simulink model "PNEUMA"  (R2023b)
settings: Solver=ode23tb  StartTime=0  StopTime=3600  FixedStep=0.001  MaxStep=time_step_new  RelTol=0.01  EnableMultiTasking=on
values from neighbouring files (symbols this model uses):
  A = 20.9    [Gas_Exchange_IC.m]    (also in getPneumonia.m = (LF1-LF2)/(1-exp(Rresolve*(t2(end)-t2(1)))))
  a1 = 0.3836    [Dissociation_Spencer_IC.m]    (also in Gas_Exchange_IC.m; Respiratory_IC.m)
  a2 = 1.819    [Dissociation_Spencer_IC.m]    (also in Gas_Exchange_IC.m; Respiratory_IC.m)
  alpha1 = 0.02598    [Dissociation_Spencer_IC.m]    (also in Gas_Exchange_IC.m; Respiratory_IC.m)
  alpha2 = 0.05591    [Dissociation_Spencer_IC.m]    (also in Gas_Exchange_IC.m; Respiratory_IC.m)
  B = 92.8    [Gas_Exchange_IC.m]    (also in getPneumonia.m = LungFunction(end)-A)
  beta1 = 0.012275    [Dissociation_Spencer_IC.m]    (also in Gas_Exchange_IC.m; Respiratory_IC.m)
  beta2 = 0.03255    [Dissociation_Spencer_IC.m]    (also in Gas_Exchange_IC.m; Respiratory_IC.m)
  C = 10570    [Gas_Exchange_IC.m]
  C1 = 9    [Dissociation_Spencer_IC.m]    (also in Gas_Exchange_IC.m; Respiratory_IC.m)
  C2 = 87.00    (= 87)    [Dissociation_Spencer_IC.m]    (also in Gas_Exchange_IC.m; Respiratory_IC.m)
  Circadian_Period = 24    [Respiratory_IC.m]    (also in State_UA_Khoo_IC.m)
  CvCO2IC = 0.5116    [Body_Khoo_IC.m]    (also in Gas_Exchange_IC.m; Respiratory_IC.m = 0.5247)
  CvO2IC = 0.1672    [Body_Khoo_IC.m]    (also in Gas_Exchange_IC.m; Respiratory_IC.m = 0.1639)
  D = -5.251    [Gas_Exchange_IC.m]
  Dead1CO2IC = 0.1020    (= 0.102)    [Dead_Space_Khoo_IC.m]    (also in Gas_Exchange_IC.m; Respiratory_IC.m = 39.5616)
  Dead1O2IC = 149.8824    [Dead_Space_Khoo_IC.m]    (also in Gas_Exchange_IC.m; Respiratory_IC.m = 104.3637)
  Dead2CO2IC = 0.5274    [Dead_Space_Khoo_IC.m]    (also in Gas_Exchange_IC.m; Respiratory_IC.m = 39.6736)
  Dead2O2IC = 149.3923    [Dead_Space_Khoo_IC.m]    (also in Gas_Exchange_IC.m; Respiratory_IC.m = 104.2258)
  Dead3CO2IC = 2.2996    [Dead_Space_Khoo_IC.m]    (also in Gas_Exchange_IC.m; Respiratory_IC.m = 39.8127)
  Dead3O2IC = 147.3503    [Dead_Space_Khoo_IC.m]    (also in Gas_Exchange_IC.m; Respiratory_IC.m = 104.0505)
  Dead4CO2IC = 8.2293    [Dead_Space_Khoo_IC.m]    (also in Gas_Exchange_IC.m; Respiratory_IC.m = 40.0061)
  Dead4O2IC = 140.5179    [Dead_Space_Khoo_IC.m]    (also in Gas_Exchange_IC.m; Respiratory_IC.m = 103.8005)
  Dead5CO2IC = 22.0757    [Dead_Space_Khoo_IC.m]    (also in Gas_Exchange_IC.m; Respiratory_IC.m = 40.3359)
  Dead5O2IC = 124.5641    [Dead_Space_Khoo_IC.m]    (also in Gas_Exchange_IC.m; Respiratory_IC.m = 103.3579)
  DtotalIC = 0.3    [NeuroMuscular_IC.m]    (also in Respiratory_IC.m = 0.32)
  E_CW = 5    [Pleural_Schuessler_IC.m]    (also in Pmus_Flow_Younes_IC.m; Resp_Mech_IC.m; Respiratory_IC.m)
  E_L = 5    [Pleural_Schuessler_IC.m]    (also in Pmus_Flow_Younes_IC.m; Resp_Mech_IC.m; Respiratory_IC.m)
  fc = 0.4/60    (= 0.00666666666667)    [Respiratory_IC.m]    (also in State_UA_Khoo_IC.m)
  fcs_max = 47.78    [Cardiovascular_IC.m]    (also in Reflex_Ursino_IC.m)
  fcs_min = 2.52    [Cardiovascular_IC.m]    (also in Reflex_Ursino_IC.m)
  fcs_zero = 25    [Respiratory_IC.m]
  FlowIC = 0    [Pmus_Flow_Younes_IC.m]    (also in Resp_Mech_IC.m; Respiratory_IC.m)
  fp_inf = 6.3    [Respiratory_IC.m]
  fp_zero = 3.2    [Respiratory_IC.m]
  fs_inf = 2.10    (= 2.1)    [Respiratory_IC.m]
  fs_zero = 16.11    [Respiratory_IC.m]
  ftbs_min = 0.1    [Cardiovascular_IC.m]    (also in SA_Node_Ursino_IC.m)
  gc = 0.008/60    (= 0.000133333333333)    [Respiratory_IC.m]    (also in State_UA_Khoo_IC.m)
  h = 0.0183    [Brain_Khoo_IC.m]    (also in Gas_Exchange_IC.m; Respiratory_IC.m)
  HP_basal = 0.58    [Cardiovascular_IC.m]    (also in SA_Node_Ursino_IC.m)
  Ic = 45    [Gas_Exchange_IC.m]    (also in Respiratory_IC.m; Vent_Drive_Khoo_IC.m)
  IpCO2 = 38    [Gas_Exchange_IC.m]    (also in Respiratory_IC.m; Vent_Drive_Khoo_IC.m)
  IpO2 = 102.4    [Gas_Exchange_IC.m]    (also in Respiratory_IC.m; Vent_Drive_Khoo_IC.m)
  K1 = 13    [Dissociation_Spencer_IC.m]    (also in Gas_Exchange_IC.m; Respiratory_IC.m)
  K2 = 194.4    [Dissociation_Spencer_IC.m]    (also in Gas_Exchange_IC.m; Respiratory_IC.m)
  k_cs = 11.758    [Cardiovascular_IC.m]    (also in Reflex_Ursino_IC.m)
  k_p = 7.06    [Respiratory_IC.m]
  k_s = 0.07    [Respiratory_IC.m]
  lambda = 863    [Gas_Exchange_IC.m]    (also in Lungs_Khoo_IC.m; Respiratory_IC.m)
  Mech_Vent_pressure = 17    [Mech_vent_test.m]
  MRbCO2 = 0.0517    [Brain_Khoo_IC.m]    (also in Gas_Exchange_IC.m; Respiratory_IC.m)
  MRCO2 = 0.0033    [Body_Khoo_IC.m]    (also in Gas_Exchange_IC.m; Respiratory_IC.m)
  MRO2 = 0.0038    [Body_Khoo_IC.m]    (also in Gas_Exchange_IC.m; Respiratory_IC.m)
  NM_block_gain = 1    [Mech_vent_test.m]
  PACO2_delayIC = 39.6041    [Cardio_Mix_Lange_IC.m]    (also in Gas_Exchange_IC.m; Respiratory_IC.m = 40.4448)
  PaCO2firstIC = 0.2150    (= 0.215)    [Cardio_Mix_Lange_IC.m]    (also in Gas_Exchange_IC.m; Respiratory_IC.m = -0.2465)
  PACO2IC = 37.1484    [Gas_Exchange_IC.m]    (also in Lungs_Khoo_IC.m; Respiratory_IC.m = 40.9432)
  PaCO2secondIC = 38.4577    [Cardio_Mix_Lange_IC.m]    (also in Gas_Exchange_IC.m; Respiratory_IC.m = 40.3928)
  PAO2_delayIC = 103.8436    [Cardio_Mix_Lange_IC.m]    (also in Gas_Exchange_IC.m; Respiratory_IC.m = 103.1223)
  PaO2firstIC = -0.2838    [Cardio_Mix_Lange_IC.m]    (also in Gas_Exchange_IC.m; Respiratory_IC.m = 0.3557)
  PAO2IC = 107.1983    [Gas_Exchange_IC.m]    (also in Lungs_Khoo_IC.m; Respiratory_IC.m = 102.5153)
  PaO2secondIC = 105.4828    [Cardio_Mix_Lange_IC.m]    (also in Gas_Exchange_IC.m; Respiratory_IC.m = 103.1435)
  PbCO2IC = 48.2858    [Brain_Khoo_IC.m]    (also in Gas_Exchange_IC.m; Respiratory_IC.m = 48.5383)
  PICO2 = 0    [Dead_Space_Khoo_IC.m]    (also in Gas_Exchange_IC.m; Respiratory_IC.m)
  PIO2 = 150    [Dead_Space_Khoo_IC.m]    (also in Gas_Exchange_IC.m; Respiratory_IC.m)
  PIO2_change = -90    [Mech_vent_test.m]    (also in Respiratory_IC.m = 0)
  Pn = 90    [Cardiovascular_IC.m]    (also in Reflex_Ursino_IC.m)
  Pt_frcIC1 = 0    [Pmus_Flow_Younes_IC.m]    (also in Resp_Mech_IC.m; Respiratory_IC.m)
  Pt_frcIC2 = 0    [Pmus_Flow_Younes_IC.m]    (also in Resp_Mech_IC.m; Respiratory_IC.m)
  QdBo = 0.8333    [Brain_Khoo_IC.m]    (also in Gas_Exchange_IC.m; Respiratory_IC.m)
  R_AW = 1.27    [Pleural_Schuessler_IC.m]    (also in Pmus_Flow_Younes_IC.m; Resp_Mech_IC.m; Respiratory_IC.m)
  R_CW = 1.03    [Pleural_Schuessler_IC.m]    (also in Pmus_Flow_Younes_IC.m; Resp_Mech_IC.m; Respiratory_IC.m)
  R_L = 1.69    [Pleural_Schuessler_IC.m]    (also in Pmus_Flow_Younes_IC.m; Resp_Mech_IC.m; Respiratory_IC.m)
  RC = 0.06    [Pleural_Schuessler_IC.m]    (also in Pmus_Flow_Younes_IC.m; Resp_Mech_IC.m; Respiratory_IC.m)
  rc = 0.2/60    (= 0.00333333333333)    [Respiratory_IC.m]    (also in State_UA_Khoo_IC.m)
  SbCO2 = 0.3600    (= 0.36)    [Brain_Khoo_IC.m]    (also in Gas_Exchange_IC.m; Respiratory_IC.m)
  SCO2 = 0.0043    [Brain_Khoo_IC.m]    (also in Gas_Exchange_IC.m; Respiratory_IC.m)
  SWAo = 0.007    [Respiratory_IC.m]    (also in State_UA_Khoo_IC.m)
  T1 = 1    [Cardio_Mix_Lange_IC.m]    (also in Gas_Exchange_IC.m; Respiratory_IC.m)
  T2 = 2    [Cardio_Mix_Lange_IC.m]    (also in Gas_Exchange_IC.m; Respiratory_IC.m)
  t_end_new = 4*24*60*60    (= 345600)    [Mech_vent_test.m]
  t_end_UA = 0    [Respiratory_IC.m]    (also in State_UA_Khoo_IC.m)
  t_Mech_Vent_duration = 0    [Mech_vent_test.m]
  t_Mech_Vent_start = 0    [Mech_vent_test.m]
  t_Mueller_duration = 0    [NeuroMuscular_IC.m]
  t_Mueller_insp = 0    [NeuroMuscular_IC.m]
  t_Mueller_start = 0    [NeuroMuscular_IC.m]
  t_NM_block_duration = 0    [Mech_vent_test.m]
  t_NM_block_start = 0    [Mech_vent_test.m]
  t_O2_duration = 0    [Mech_vent_test.m]    (also in Respiratory_IC.m)
  t_O2_start = 0    [Mech_vent_test.m]    (also in Respiratory_IC.m)
  t_start_new = 0    [Mech_vent_test.m]
  t_start_UA = 0    [Respiratory_IC.m]    (also in State_UA_Khoo_IC.m)
  t_valsalva_duration = 0    [NeuroMuscular_IC.m]
  t_valsalva_insp = 0    [NeuroMuscular_IC.m]
  t_valsalva_start = 0    [NeuroMuscular_IC.m]
  time_step = time_step    [acquire_data.m]    (also in acquire_data_save.m)
  VC = 5    [Pmus_Flow_Younes_IC.m]    (also in Resp_Mech_IC.m; Respiratory_IC.m)
  Vdead1 = 0.03    [Dead_Space_Khoo_IC.m]    (also in Gas_Exchange_IC.m; Respiratory_IC.m)
  Vdead2 = 0.03    [Dead_Space_Khoo_IC.m]    (also in Gas_Exchange_IC.m; Respiratory_IC.m)
  Vdead3 = 0.03    [Dead_Space_Khoo_IC.m]    (also in Gas_Exchange_IC.m; Respiratory_IC.m)
  Vdead4 = 0.03    [Dead_Space_Khoo_IC.m]    (also in Gas_Exchange_IC.m; Respiratory_IC.m)
  Vdead5 = 0.03    [Dead_Space_Khoo_IC.m]    (also in Gas_Exchange_IC.m; Respiratory_IC.m)
  Ventilator_rate = 12    [Mech_vent_test.m]
  VTCO2 = 15    [Body_Khoo_IC.m]    (also in Gas_Exchange_IC.m; Respiratory_IC.m)
  VtIC = 0    [Pmus_Flow_Younes_IC.m]    (also in Resp_Mech_IC.m; Respiratory_IC.m)
  VTO2 = 6    [Body_Khoo_IC.m]    (also in Gas_Exchange_IC.m; Respiratory_IC.m)
  Z = 0.0227    [Dissociation_Spencer_IC.m]    (also in Gas_Exchange_IC.m; Respiratory_IC.m)
undefined symbols (not defined in the file or in its folder): A_0_ua, alpha_E_FFA_Heart, alpha_E_FFA_muscle, alpha_E_GLC_Heart, alpha_E_GLC_muscle, alpha_E_GLY_muscle, alpha_E_PYR_muscle, alpha_E_TGL_adipose, alpha_E_TGL_GI, alpha_E_TGL_Heart, alpha_E_TGL_muscle, Arousal_UAIC, C_ua_awake, Cbp, Cbv, Ce_0, Cep, Cev, Chp, Chv, Cla, Clamp_class, Cmp, Cmv, Cpa, CPAP_pressure, Cpp, Cpv, Cra, Csa, Csp, Csv, CvbO2_n, CvhO2_n, CvmO2_n, DAY, delay, DietBlock, Dx, Fb, fchemo_max, fchemo_min, fchemoIC, flsIC, Ftas_I0, ftas_min, ftas_r0, FVC_activation, gain_E, Gamma, Gas_sleep, Gas_sleepM, Gb, Gblock, GbO2, Gbs_sleep, gcc_sa, gcc_sb, gcc_sp, Gclamp ... (+144)
libraries: simulink x4, dspstat3 x4, simulink_extras x2
(part 3 of 8)

== system PNEUMA/FVC + Valsalva + Mueller maneuvers/MEFV Operation ==
  Fcn1 : Fcn  Expr=1-u
  Mux2 : Mux  Inputs=3
  Step : Step  Time=begin_time  SampleTime=0
  Step1 : Step  Time=begin_time+duration_time  After=-1  SampleTime=0
  Step3 : Step  Time=begin_time+insp_period  After=-1  SampleTime=0
  Step5 : Step  Time=begin_time+insp_period  After=-1  SampleTime=0
  Step7 : Step  Time=begin_time+0.01  After=-1  SampleTime=0
  Step8 : Step  Time=begin_time+insp_period  SampleTime=0
  Step9 : Step  Time=begin_time+duration_time  After=-1  SampleTime=0
  Sum{,1..4} (5 alike) : Sum  Inputs=|++  InputSameDT=on  SaturateOnIntegerOverflow=on  OutDataTypeStr=Inherit: Same as first input
  duration : Outport
  FVC_rhythm : Outport  Port=2
  FVC_resp_mech : Outport  Port=3
  wires:
  Fcn1/1 -> duration/1
  Sum4/1 -> FVC_resp_mech/1
  Step8/1 -> Sum4/1
  Mux2/1 -> FVC_rhythm/1
  Sum3/1 -> Mux2/3
  Step7/1 -> Sum3/2
  Sum2/1 -> Mux2/2
  Step5/1 -> Sum2/2
  Sum1/1 -> Mux2/1
  Step3/1 -> Sum1/2
  Sum/1 -> Fcn1/1
  Step1/1 -> Sum/2
  Step/1 -> Sum/1, Sum1/1, Sum2/1, Sum3/1
  Step9/1 -> Sum4/2

== system PNEUMA/FVC + Valsalva + Mueller maneuvers/Mueller Operation ==
  Fcn1 : Fcn  Expr=1-u
  Fcn2 : Fcn  Expr=1-u
  Mux2 : Mux  Inputs=3
  Step : Step  Time=begin_time  SampleTime=0
  Step1 : Step  Time=begin_time+duration_time  After=-1  SampleTime=0
  Step3 : Step  Time=begin_time+insp_period  After=-1  SampleTime=0
  Step5 : Step  Time=begin_time+insp_period  After=-1  SampleTime=0
  Step7 : Step  Time=begin_time+0.01  After=-1  SampleTime=0
  Step9 : Step  Time=begin_time+insp_period+0.5  After=-1  SampleTime=0
  Sum{,1..4} (5 alike) : Sum  Inputs=|++  InputSameDT=on  SaturateOnIntegerOverflow=on  OutDataTypeStr=Inherit: Same as first input
  duration : Outport
  mueller_rhythm : Outport  Port=2
  muller_resp_mech : Outport  Port=3
  wires:
  Fcn2/1 -> muller_resp_mech/1
  Fcn1/1 -> duration/1
  Step/1 -> Sum/1, Sum1/1, Sum2/1, Sum3/1, Sum4/1
  Step1/1 -> Sum/2
  Sum/1 -> Fcn1/1
  Step3/1 -> Sum1/2
  Sum1/1 -> Mux2/1
  Step5/1 -> Sum2/2
  Sum2/1 -> Mux2/2
  Step7/1 -> Sum3/2
  Sum3/1 -> Mux2/3
  Mux2/1 -> mueller_rhythm/1
  Step9/1 -> Sum4/2
  Sum4/1 -> Fcn2/1

== system PNEUMA/FVC + Valsalva + Mueller maneuvers/Valsalva Operation ==
  Fcn1 : Fcn  Expr=1-u
  Mux2 : Mux  Inputs=3
  Step : Step  Time=begin_time  SampleTime=0
  Step1 -(TTmean-TImean) : Step  Time=begin_time+duration_time  After=-1  SampleTime=0
  Step3 : Step  Time=begin_time+insp_period  After=-1  SampleTime=0
  Step5 : Step  Time=begin_time+insp_period  After=-1  SampleTime=0
  Step7 : Step  Time=begin_time+0.01  After=-1  SampleTime=0
  Step8 : Step  Time=begin_time+insp_period  SampleTime=0
  Step9 : Step  Time=begin_time+duration_time  After=-1  SampleTime=0
  Sum{,1..4} (5 alike) : Sum  Inputs=|++  InputSameDT=on  SaturateOnIntegerOverflow=on  OutDataTypeStr=Inherit: Same as first input
  duration : Outport
  valsalva_rhythm : Outport  Port=2
  valsalva_resp_mech : Outport  Port=3
  wires:
  Fcn1/1 -> duration/1
  Sum4/1 -> valsalva_resp_mech/1
  Step8/1 -> Sum4/1
  Mux2/1 -> valsalva_rhythm/1
  Sum3/1 -> Mux2/3
  Step7/1 -> Sum3/2
  Sum2/1 -> Mux2/2
  Step5/1 -> Sum2/2
  Sum1/1 -> Mux2/1
  Step3/1 -> Sum1/2
  Sum/1 -> Fcn1/1
  Step1 -(TTmean-TImean)/1 -> Sum/2
  Step/1 -> Sum/1, Sum1/1, Sum2/1, Sum3/1
  Step9/1 -> Sum4/2

== system PNEUMA/Metabolic Control/Display & Storage ==
  note: Sample Rate: Default
  I(t)_in : Inport
  G(t) : Inport  Port=2
  I(t) : Inport  Port=3
  F(t) : Inport  Port=4
  E(t) : Inport  Port=5
  Gin : Inport  Port=6
  Gclamp_in : Inport  Port=7
  Main Display : Scope  NumInputPorts=6
  Mux : Mux  Inputs=7
  Saving G_I_FFA : Subsystem
  tag scope: Epinephrine=global, FFA=global, Glucose=global, GlucoseInput=global, Insulin=global
  wires:
  G(t)/1 -> Main Display/1, Mux/1, [Glucose]
  I(t)/1 -> Main Display/2, Mux/2, [Insulin]
  F(t)/1 -> Mux/3, Main Display/3, [FFA]
  E(t)/1 -> Mux/4, Main Display/4, [Epinephrine]
  Gin/1 -> Mux/5, [GlucoseInput], Main Display/5
  I(t)_in/1 -> Mux/6
  Mux/1 -> Saving G_I_FFA/1(In1)
  Gclamp_in/1 -> Main Display/6, Mux/7

== system PNEUMA/Metabolic Control/Epinephrine Regulation on Heart and Muscle ==
  note: (micronmol/min)
  note: (micronmol/min)
  note: (micronmol/min)
  Ftas_r : Inport
  SI : Inport  Port=2
  REM : Inport  Port=3
  1microMol = 1e6 pMol : Gain  Gain=1e6  SaturateOnIntegerOverflow=on  OutDataTypeStr=Inherit: Same as input  ParamDataTypeStr=Inherit: Same as input
  Demux : Demux
  Demux1 : Demux  Outputs=5
  EPI Modulation : Scope  NumInputPorts=10
  Epi Dynamics : Subsystem
  Epi Modulation : Subsystem
  FLux Scope : Scope  NumInputPorts=4
  Subtract : Sum  Inputs=-+
  Subtract1 : Sum  Inputs=-+
  "Epi_Heart Glucose " : Outport
  Epi_Muscle Glucose : Outport  Port=2
  "Epi_Heart FFA " : Outport  Port=3
  Epi_Muscle FFA : Outport  Port=4
  Epi_GI FFA : Outport  Port=5
  Epinephrine Amount Ce(t) : Outport  Port=6
  W_alphaSYMP : Outport  Port=7
  wires:
  Epi Dynamics/1(Ce(t)) -> 1microMol = 1e6 pMol/1
  Epi Modulation/1(Epi on Heart) -> FLux Scope/1
  Epi Modulation/2(Epi on Muscle) -> FLux Scope/2
  Epi Modulation/3(Epi on GI) -> FLux Scope/3, EPI Modulation/10, Epi_GI FFA/1
  Epi Modulation/4(Epi on adipose) -> FLux Scope/4
  1microMol = 1e6 pMol/1 -> Epi Modulation/1(Ce(t)), Epinephrine Amount Ce(t)/1
  Epi Modulation/5(4Fluxes of Epi in Heart) -> Demux/1
  Epi Modulation/6(5Fluxes of Epi in Muscle) -> Demux1/1
  Demux/1 -> EPI Modulation/1, "Epi_Heart Glucose "/1
  Demux/2 -> EPI Modulation/2
  Demux/3 -> EPI Modulation/3, Subtract/1
  Demux/4 -> EPI Modulation/4, Subtract/2
  Demux1/1 -> EPI Modulation/5, Epi_Muscle Glucose/1
  Demux1/2 -> EPI Modulation/6
  Demux1/3 -> EPI Modulation/7
  Demux1/4 -> EPI Modulation/8, Subtract1/1
  Demux1/5 -> EPI Modulation/9, Subtract1/2
  Subtract/1 -> "Epi_Heart FFA "/1
  Subtract1/1 -> Epi_Muscle FFA/1
  Ftas_r/1 -> Epi Dynamics/1(Ftas_r)
  SI/1 -> Epi Dynamics/2(SI)
  REM/1 -> Epi Dynamics/3(REM)
  Epi Dynamics/2(W_alphaSYMP) -> W_alphaSYMP/1

== system PNEUMA/Metabolic Control/Gain ==
  In1 : Inport
  In2 : Inport  Port=2
  In3 : Inport  Port=3
  In4 : Inport  Port=4
  In5 : Inport  Port=5
  Subtract1 : Sum
  Subtract2 : Sum  Inputs=+++
  micromol to mg : Gain  Gain=0.0018*gain_E
  micromol to mg1 : Gain  Gain=0.01*gain_E
  G_E : Outport
  F_E : Outport  Port=2
  wires:
  Subtract1/1 -> micromol to mg/1  "Glucose Input"
  Subtract2/1 -> micromol to mg1/1  "FFA Input"
  In1/1 -> Subtract1/1
  micromol to mg/1 -> G_E/1  "Glucose Input"
  In2/1 -> Subtract1/2
  In3/1 -> Subtract2/1
  In4/1 -> Subtract2/2
  micromol to mg1/1 -> F_E/1
  In5/1 -> Subtract2/3

== system PNEUMA/Metabolic Control/Glucose Insulin Interventions ==
  note: 1-IVGTT (1hr only)
      | 2-Glucose Clamps
  G(t) : Inport
  1-Hyper&2-Norm_Hypo : Constant  Value=Clamp_class
  GI_CTRL : Constant  Value=GI_CTRL
  Gblock : Gain  Gain=0
  Hyper/Eu/Hypo glycemic Clamp (step by step) : Subsystem
  IVGTT : Subsystem  mask{begin_time=0, end_time=1*60, init_value=330*70/70, end_value=0}
      mask prompts: begin_time "begin time"; end_time "end time"; init_value "initial value"; end_value "end value"
      mask Display: disp('IVGTT')
  Iblock : Gain  Gain=0
  Insulin Pump Euglycemic Clamp : Subsystem
  Multiport Switch : MultiPortSwitch  Inputs=2  SaturateOnIntegerOverflow=off  InputSameDT=off
  Glu_in(t) : Outport
  Gclamp_in(t) : Outport  Port=2
  InsPump_in(t) : Outport  Port=3
  wires:
  IVGTT/1(Out1) -> Multiport Switch/2
  Multiport Switch/1 -> Gblock/1
  GI_CTRL/1 -> Multiport Switch/1
  Insulin Pump Euglycemic Clamp/1(Out1) -> Iblock/1
  Hyper/Eu/Hypo glycemic Clamp (step by step)/1(u(t)) -> Multiport Switch/3
  1-Hyper&2-Norm_Hypo/1 -> Hyper/Eu/Hypo glycemic Clamp (step by step)/2(Clamp Classifier)
  G(t)/1 -> Hyper/Eu/Hypo glycemic Clamp (step by step)/1(G(t))
  Gblock/1 -> Glu_in(t)/1
  Hyper/Eu/Hypo glycemic Clamp (step by step)/2(Glu_In Rate) -> Gclamp_in(t)/1
  Iblock/1 -> InsPump_in(t)/1

== system PNEUMA/Metabolic Control/Glucose-Insulin-FFA Minimal Model ==
  note: Remote
      | Insulin
      | X(t)
  u1(t) : Inport
  u2(t) : Inport  Port=2
  u3(t) : Inport  Port=3
  W_alphaSYMP : Inport  Port=4
  2*Fcn+2 : Fcn  Expr=2*Ftas_I0* ( exp((u-Ib)/k_isc_I) -1) / (1+ exp((u-Ib)/k_isc_I) )+2
  FFA Dynamics_LC : Subsystem
  Gain1 : Gain  Gain=1/tao_I
  Glucose Dynamics_LC : Subsystem
  Insulin Dynamics _ B&P : Subsystem
  Integrator1 : Integrator
  Mux : Mux  Inputs=2
  Remote Compartment p3 / (s + p2)1 : Subsystem
  Remote Ins_FFA pF3 / (s + pF2) : Subsystem
  Saving deltaFtas_WalphaSYMP : Subsystem
  Subsystem : Subsystem
  Sum2 : Sum  Inputs=-+  InputSameDT=on  SaturateOnIntegerOverflow=on  OutDataTypeStr=Inherit: Same as first input
  "Plasma Glucose Concn, G(t)" : Outport
  "Plasma Insulin Concn, I(t)" : Outport  Port=2
  "Plasma FFA Concn, F(t)" : Outport  Port=3
  DeltaFtas : Outport  Port=4
  wires:
  Remote Compartment p3 / (s + p2)1/1(X(t)) -> Glucose Dynamics_LC/3(X(t))
  u3(t)/1 -> FFA Dynamics_LC/3(u3(t))
  u2(t)/1 -> Glucose Dynamics_LC/1(u2(t))
  u1(t)/1 -> Insulin Dynamics _ B&P/2(u1(t))
  FFA Dynamics_LC/1(F(t)) -> "Plasma FFA Concn, F(t)"/1, Subsystem/1(F(t))
  Subsystem/1(Z(t)) -> Glucose Dynamics_LC/2(Z(t))  "Remote FFA  Z(t)"
  Insulin Dynamics _ B&P/1(I(t)) -> "Plasma Insulin Concn, I(t)"/1, 2*Fcn+2/1, Remote Compartment p3 / (s + p2)1/1(I(t)), Remote Ins_FFA pF3 / (s + pF2)/1(I(t))
  Remote Ins_FFA pF3 / (s + pF2)/1(Y(t)) -> FFA Dynamics_LC/2(Y(t))
  Sum2/1 -> Gain1/1
  Integrator1/1 -> Sum2/1, Mux/1, DeltaFtas/1
  Gain1/1 -> Integrator1/1
  2*Fcn+2/1 -> Sum2/2
  Glucose Dynamics_LC/1(G(t)) -> "Plasma Glucose Concn, G(t)"/1, Insulin Dynamics _ B&P/1(G(t)), FFA Dynamics_LC/1(G(t))
  W_alphaSYMP/1 -> Mux/2
  Mux/1 -> Saving deltaFtas_WalphaSYMP/1(In1)

== system PNEUMA/Metabolic Control/Insulin Clamp ==
  note: 90-minute Insulin Pump (through 4 steps injections)
  Add : Sum  Inputs=+++++
  Step : Step  Time=2*60+delay+60*2*60  After=step_u1  SampleTime=0
  Step1 : Step  Time=4*60+delay+60*2*60  After=step_u1  SampleTime=0
  Step2 : Step  Time=6*60+delay+60*2*60  After=step_u1  SampleTime=0
  Step3 : Step  Time=8*60+delay+60*2*60  After=step_u1  SampleTime=0
  Step4 : Step  Time=90*60+delay+60*2*60  After=-4*step_u1*Ins_shutdown  SampleTime=0
  Insulin Input : Outport
  wires:
  Step/1 -> Add/1
  Step1/1 -> Add/2
  Step3/1 -> Add/4
  Step2/1 -> Add/3
  Add/1 -> Insulin Input/1
  Step4/1 -> Add/5

== system PNEUMA/Respiratory System/Gas Exchange ==
  Vt - Tidal Volume : Inport
  SI Sleep Wake State Index : Inport  Port=2
  Air Flow : Inport  Port=3
  Blood Flow : Inport  Port=4
  BODY TISSUES COMPARTMENT : Subsystem
  BRAIN COMPARTMENT : Subsystem
  Blood Flow to Tissues : Gain  Gain=0.85  SaturateOnIntegerOverflow=on  OutDataTypeStr=Inherit: Same as input  ParamDataTypeStr=Inherit: Same as input
  Cardiovascular Mixing and Convection : Subsystem
  DEAD SPACE : Subsystem
  Dissociation : Subsystem
  GAS EXCHANGE IN THE LUNGS : Subsystem
  Lung-Chemo Volume : Constant  Value=0.588
  VARIATION OF CEREBRAL BLOOD FLOW W/ PaCO2 Fcn : Fcn  Expr=(sqrt(abs( ((1+(u - 40) * .03 ) * (-QdBo))^2 - ( MRbCO2-h) * 4*0.03*QdBo/SCO2 ) )- (1+(u - 40) * .03 ) * (-QdBo)) *0.5
  PaCO2 : Outport
  PaO2 : Outport  Port=2
  SAO2 : Outport  Port=3
  PbCO2 : Outport  Port=4
  CaO2 : Outport  Port=5
  tag scope: PaCO2=global, PaO2=global, SAO2=global
  wires:
  SI Sleep Wake State Index/1 -> BODY TISSUES COMPARTMENT/1(SI Sleep Wake State Index), BRAIN COMPARTMENT/3(SI Sleep Wake State Index)
  Cardiovascular Mixing and Convection/1(PaCO2) -> BRAIN COMPARTMENT/2(PaCO2), [PaCO2], PaCO2/1  "PaCO2"
  BRAIN COMPARTMENT/1(PbCO2) -> PbCO2/1, VARIATION OF CEREBRAL BLOOD FLOW W/ PaCO2 Fcn/1  "PbCO2"
  DEAD SPACE/1(Pd5CO2) -> GAS EXCHANGE IN THE LUNGS/3(Pd5CO2)
  DEAD SPACE/2(Pd5O2) -> GAS EXCHANGE IN THE LUNGS/4(Pd5O2)
  GAS EXCHANGE IN THE LUNGS/2(PAO2) -> DEAD SPACE/2(PAO2), Cardiovascular Mixing and Convection/3(PAO2), Dissociation/2(PAO2)  "PAO2"
  Vt - Tidal Volume/1 -> GAS EXCHANGE IN THE LUNGS/6(Vt - Tidal Volume)
  Air Flow/1 -> DEAD SPACE/3(Flow), GAS EXCHANGE IN THE LUNGS/5(Flow)
  VARIATION OF CEREBRAL BLOOD FLOW W/ PaCO2 Fcn/1 -> BRAIN COMPARTMENT/1(Qb)  "Qb"
  GAS EXCHANGE IN THE LUNGS/1(PACO2) -> DEAD SPACE/1(PACO2), Cardiovascular Mixing and Convection/2(PACO2), Dissociation/1(PACO2)  "PACO2"
  Lung-Chemo Volume/1 -> Cardiovascular Mixing and Convection/1(Lung-Chemoreceptor Delay Volume)
  Blood Flow/1 -> Blood Flow to Tissues/1, GAS EXCHANGE IN THE LUNGS/7("Q "), Cardiovascular Mixing and Convection/4(Q)
  Cardiovascular Mixing and Convection/2(PaO2) -> [PaO2], PaO2/1  "PaO2"
  Blood Flow to Tissues/1 -> BODY TISSUES COMPARTMENT/4("Qt ")
  Dissociation/1(CaCO2) -> GAS EXCHANGE IN THE LUNGS/1(CaCO2), BODY TISSUES COMPARTMENT/2(CaCO2)
  Dissociation/3(CaO2) -> GAS EXCHANGE IN THE LUNGS/9(CaO2), CaO2/1, BODY TISSUES COMPARTMENT/3(CaO2)
  Dissociation/2(SAO2) -> [SAO2], SAO2/1
  BODY TISSUES COMPARTMENT/1(CvCO2) -> GAS EXCHANGE IN THE LUNGS/2(CVCO2)
  BODY TISSUES COMPARTMENT/2(CvO2) -> GAS EXCHANGE IN THE LUNGS/8(CVO2)

== system PNEUMA/Respiratory System/Modified Upper Airway Conductance ==
  Fcn1 : Fcn  Expr=1-u
  Fcn2 : Fcn  Expr=(u(1)==0)*1+(u(1)==1)*u(2)
  Fcn3 : Fcn  Expr=(u(1)==0)*1+(u(1)==1)*u(2)
  Memory : Memory
  Mux1 : Mux  Inputs=2
  Mux3 : Mux  Inputs=2
  Product2 : Product  Inputs=***  InputSameDT=on  SaturateOnIntegerOverflow=on  OutDataTypeStr=Inherit: Same as first input
  Sum : Sum
  Terminator : Terminator
  UA_blocker : Gain  Gain=0  SaturateOnIntegerOverflow=on  OutDataTypeStr=Inherit: Same as input  ParamDataTypeStr=Inherit: Same as input
  UPC Scope : Scope  NumInputPorts=4
  Upper Airway Blockage : Subsystem  mask{begin_time=t_start_UA, end_time=t_end_UA}
      mask prompts: begin_time "pulse begin"; end_time "pulse end"
      mask Display: disp('pulse')
  func : Fcn  Expr=1-u
  modified upper airway : Outport
  tag scope: upper_airway_blockage_duration=global
  wires:
  Upper Airway Blockage/1(Out1) -> func/1
  [Valsalva_resp_mech] -> Fcn1/1
  UA_blocker/1 -> [upper_airway_blockage_duration], Sum/1
  [CONDua] -> Product2/1, UPC Scope/3
  Product2/1 -> UPC Scope/2, Sum/2
  func/1 -> UA_blocker/1
  [Mueller_activation] -> Mux3/1
  [Mueller_resp_mech] -> Mux3/2
  Mux3/1 -> Fcn2/1
  Fcn2/1 -> Product2/2
  [Valsalva_activation] -> Mux1/1
  Mux1/1 -> Fcn3/1
  Fcn1/1 -> Mux1/2
  Fcn3/1 -> UPC Scope/4, Terminator/1, Product2/3
  Memory/1 -> modified upper airway/1, UPC Scope/1
  Sum/1 -> Memory/1

== system PNEUMA/Respiratory System/Respiratory_Mechanics ==
  "RespMus Drive " : Inport
  Respiratory Conductance : Inport  Port=2
  "PE " : Inport  Port=3
  "Pao " : Inport  Port=4
  Step Size : Inport  Port=5
  Enable : EnablePort  StatesWhenEnabling=reset  ZeroCross=off
  External Pressure Gain : Gain  Gain=0.1  SaturateOnIntegerOverflow=on  OutDataTypeStr=Inherit: Same as input  ParamDataTypeStr=Inherit: Same as input
  Pleural Pressure Saturation : Saturate  UpperLimit=160  LowerLimit=-40  LinearizeAsGain=off  ZeroCross=off
  Pleural_Pressure1 : Subsystem
  Respiratory Muscles Activity1 : Subsystem
  Vt - Tidal Volume : Outport  InitialOutput=[0]
  Respiratory Flow : Outport  Port=2  InitialOutput=[0]
  "Ppl " : Outport  Port=3  InitialOutput=[0]
  wires:
  "PE "/1 -> Respiratory Muscles Activity1/2(PE)
  "RespMus Drive "/1 -> Respiratory Muscles Activity1/1(RespMus Drive)
  Respiratory Conductance/1 -> Respiratory Muscles Activity1/3("cond ")
  Respiratory Muscles Activity1/3(Pmus) -> Pleural_Pressure1/3(Pmus)
  "Pao "/1 -> External Pressure Gain/1
  External Pressure Gain/1 -> Pleural_Pressure1/4("Pao "), Respiratory Muscles Activity1/5(Pao)
  Respiratory Muscles Activity1/2(Vt) -> Pleural_Pressure1/2(Vt), Vt - Tidal Volume/1  "Vt Tidal Volume"
  Respiratory Muscles Activity1/1(Respiratory Flow) -> Pleural_Pressure1/1(Respiratory Flow), Respiratory Flow/1  "Flow"
  Step Size/1 -> Respiratory Muscles Activity1/4(Step Size)
  Pleural_Pressure1/1("Pleural Pressure (Ppl) ") -> Pleural Pressure Saturation/1
  Pleural Pressure Saturation/1 -> "Ppl "/1

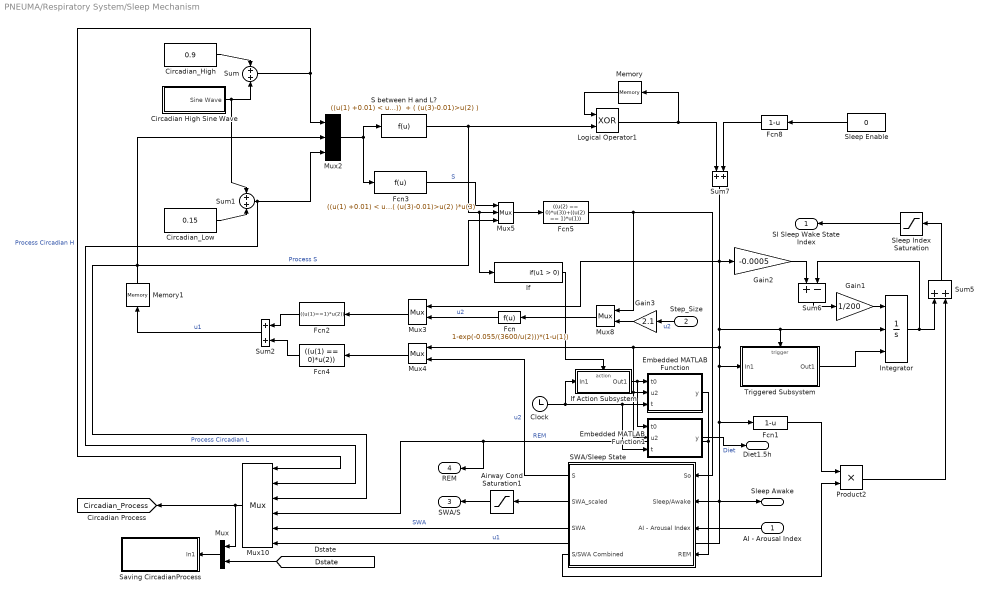
== system PNEUMA/Respiratory System/Sleep Mechanism ==
  AI - Arousal Index : Inport
  Step_Size : Inport  Port=2
  Airway Cond Saturation1 : Saturate  UpperLimit=1  LowerLimit=0
  Circadian High Sine Wave : Subsystem
  Circadian_High : Constant  Value=0.9
  Circadian_Low : Constant  Value=0.15
  Clock : Clock
  Embedded MATLAB Function : MATLAB Function  TreatAsAtomicUnit=on
  Embedded MATLAB Function1 : MATLAB Function  TreatAsAtomicUnit=on
  Fcn : Fcn  Expr=1-exp(-0.055/(3600/u(2)))*(1-u(1))
  Fcn1 : Fcn  Expr=1-u
  Fcn2 : Fcn  Expr=((u(1)==1)*u(2))
  Fcn3 : Fcn  Expr=((u(1) +0.01) < u(2)) * u(1) + ( (u(3)-0.01)>u(2) )*u(3)
  Fcn4 : Fcn  Expr=((u(1) == 0)*u(2))
  Fcn5 : Fcn  Expr=((u(2) == 0)*u(3))+((u(2) == 1)*u(1))
  Fcn8 : Fcn  Expr=1-u
  Gain1 : Gain  Gain=1/200  SaturateOnIntegerOverflow=on  OutDataTypeStr=Inherit: Same as input  ParamDataTypeStr=Inherit: Same as input
  Gain2 : Gain  Gain=-0.0005  SaturateOnIntegerOverflow=on  OutDataTypeStr=Inherit: Same as input  ParamDataTypeStr=Inherit: Same as input
  Gain3 : Gain  Gain=2.1  SaturateOnIntegerOverflow=on  OutDataTypeStr=Inherit: Same as input  ParamDataTypeStr=Inherit: Same as input
  If : If  ShowElse=off
  If Action Subsystem : Subsystem  TreatAsAtomicUnit=on
  Integrator : Integrator  ExternalReset=rising  InitialConditionSource=external  InitialCondition=1
  Logical Operator1 : Logic  Operator=XOR
  Memory : Memory  InitialCondition=1  InheritSampleTime=on
  Memory1 : Memory  InitialCondition=1  InheritSampleTime=on
  Mux{,3..4,8} (4 alike) : Mux  Inputs=2
  Mux10 : Mux  Inputs=6
  Mux2 : Mux  Inputs=3
  Mux5 : Mux  Inputs=3
  Product2 : Product  InputSameDT=on  SaturateOnIntegerOverflow=on  OutDataTypeStr=Inherit: Same as first input
  S between H and L? : Fcn  Expr="((u(1) +0.01) < u(2))  + ( (u(3)-0.01)>u(2) )"
  SWA/Sleep State : Subsystem
  Saving CircadianProcess : Subsystem
  Sleep Enable : Constant  Value=0
  Sleep Index Saturation : Saturate  UpperLimit=1  LowerLimit=0
  Sum{,1..2,5,7} (5 alike) : Sum  InputSameDT=on  SaturateOnIntegerOverflow=on  OutDataTypeStr=Inherit: Same as first input
  Sum6 : Sum  Inputs=+-  InputSameDT=on  SaturateOnIntegerOverflow=on  OutDataTypeStr=Inherit: Same as first input
  Triggered Subsystem : Subsystem  TreatAsAtomicUnit=on
  SI Sleep Wake State Index : Outport
  Sleep Awake : Outport  Port=2
  SWA/S : Outport  Port=3
  REM : Outport  Port=4
  Diet1.5h : Outport  Port=5
  tag scope: Circadian_Process=global
  wires:
  AI - Arousal Index/1 -> SWA/Sleep State/3(AI - Arousal Index)
  Circadian_High/1 -> Sum/1
  Circadian High Sine Wave/1(Sine Wave) -> Sum/2, Sum1/1
  Circadian_Low/1 -> Sum1/2
  Sum/1 -> Mux2/1, Mux10/1  "Process Circadian H"
  Sum1/1 -> Mux2/3, Mux10/2  "Process Circadian L"
  Memory/1 -> Logical Operator1/1
  Logical Operator1/1 -> Memory/1, Sum7/1
  Fcn3/1 -> Mux5/1  "S"
  Fcn2/1 -> Sum2/1
  Sum2/1 -> Memory1/1  "u1"
  Fcn/1 -> Mux3/2  "u2"
  SWA/Sleep State/1(S) -> Mux4/2  "u2"
  Mux5/1 -> Fcn5/1
  Mux3/1 -> Fcn2/1
  Mux4/1 -> Fcn4/1
  Fcn5/1 -> SWA/Sleep State/1(So), Mux8/1
  Mux8/1 -> Fcn/1
  Step_Size/1 -> Gain3/1  "u2"
  SWA/Sleep State/2(SWA_scaled) -> Airway Cond Saturation1/1
  Airway Cond Saturation1/1 -> SWA/S/1
  Mux10/1 -> [Circadian_Process], Mux/1
  SWA/Sleep State/3(SWA) -> Mux10/5  "SWA"
  SWA/Sleep State/4(S/SWA Combined) -> Product2/2
  Fcn1/1 -> Product2/1
  Sum5/1 -> Sleep Index Saturation/1
  Product2/1 -> Sum5/2
  Sleep Index Saturation/1 -> SI Sleep Wake State Index/1
  Sum7/1 -> Mux3/1, Triggered Subsystem/Trigger, Integrator/2, Fcn1/1, Sleep Awake/1, SWA/Sleep State/2(Sleep/Awake), Mux10/6, Triggered Subsystem/1(In1), Mux4/1, Embedded MATLAB Function/2(u2), Embedded MATLAB Function1/2(u2), Gain2/1  "u1"
  Integrator/1 -> Sum5/1, Sum6/2
  Triggered Subsystem/1(Out1) -> Integrator/3
  Gain2/1 -> Sum6/1
  Sum6/1 -> Gain1/1
  Gain1/1 -> Integrator/1
  Fcn8/1 -> Sum7/2
  Memory1/1 -> Mux5/3, Mux10/3, Mux2/2  "Process S"
  Mux2/1 -> Fcn3/1, S between H and L?/1
  S between H and L?/1 -> Logical Operator1/2, Mux5/2, If/1
  Gain3/1 -> Mux8/2
  If Action Subsystem/1(Out1) -> Embedded MATLAB Function/1(t0), Embedded MATLAB Function1/1(t0)
  If/1 -> If Action Subsystem/Action
  Fcn4/1 -> Sum2/2
  Clock/1 -> If Action Subsystem/1(In1), Embedded MATLAB Function/3(t), Embedded MATLAB Function1/3(t)
  Embedded MATLAB Function/1(y) -> SWA/Sleep State/4(REM), Mux10/4, REM/1  "REM"
  Sleep Enable/1 -> Fcn8/1
  [Dstate] -> Mux/2
  Mux/1 -> Saving CircadianProcess/1(In1)
  Embedded MATLAB Function1/1(y) -> Diet1.5h/1  "Diet"

== system PNEUMA/Respiratory System/Upper_Airway_Mechanism ==
  SI Sleep Wake State Index : Inport
  Variable Respiratory Rhythm : Inport  Port=2
  Total Ventilatory Drive : Inport  Port=3
  extern pressure : Inport  Port=4
  Pleural Pressure : Inport  Port=5
  Respiratory Flow Lower Airways : Inport  Port=6
  Tidal Volume : Inport  Port=7
  Sleep/Awake : Inport  Port=8
  SWA/S : Inport  Port=9
  Arousal Threshold : Fcn  Expr=(u(1) > (Ivent - Ivent*0.3*(1-u(2) ) ) )
  Mux : Mux  Inputs=2
  State-dependent Upper Airway model : Subsystem
  Upper_Airway_Model : Subsystem  TreatAsAtomicUnit=on
  AI - Arousal Index : Outport
  "Airway Cond Percentage " : Outport  Port=2
  wires:
  SI Sleep Wake State Index/1 -> Upper_Airway_Model/1(SI Sleep Wake State Index), State-dependent Upper Airway model/1(SI Sleep Wake State Index)
  extern pressure/1 -> State-dependent Upper Airway model/3(External Pressure)
  SWA/S/1 -> Mux/2, State-dependent Upper Airway model/5(SWA/S)
  Total Ventilatory Drive/1 -> Upper_Airway_Model/6(Total Ventilatory Drive), Mux/1  "Ventilatory Drive"
  Sleep/Awake/1 -> State-dependent Upper Airway model/4(Sleep/Awake), Upper_Airway_Model/7(Sleep/awake)
  Upper_Airway_Model/1("Y_ua Upper Airway Conductance ") -> "Airway Cond Percentage "/1  "State Dependent Conductance"
  Variable Respiratory Rhythm/1 -> Upper_Airway_Model/2(Respiratory Rhythm)
  Respiratory Flow Lower Airways/1 -> Upper_Airway_Model/3(Q_total Total Respiratory Flow Airways)
  Pleural Pressure/1 -> Upper_Airway_Model/4(Pleural Pressure)
  Tidal Volume/1 -> Upper_Airway_Model/5(Tidal Volume)
  [Breathing_Enable] -> Upper_Airway_Model/Enable
  Mux/1 -> Arousal Threshold/1
  Arousal Threshold/1 -> AI - Arousal Index/1, State-dependent Upper Airway model/2(AI - Arousal Index)

== system PNEUMA/Ventilator/Saving CONTROLLER ==
  In1 : Inport
  Clock : Clock
  Gain : Gain  Gain=1/(3600*24*DAY)
  Rounding Function : Rounding
  Switch Case : SwitchCase  CaseConditions={0,1,2,3,4,5,6,7,8}  SampleTime=sampletime
  Switch Case Action Subsystem : Subsystem  TreatAsAtomicUnit=on
  Switch Case Action Subsystem1 : Subsystem  TreatAsAtomicUnit=on
  Switch Case Action Subsystem2 : Subsystem  TreatAsAtomicUnit=on
  Switch Case Action Subsystem3 : Subsystem  TreatAsAtomicUnit=on
  Switch Case Action Subsystem4 : Subsystem  TreatAsAtomicUnit=on
  Switch Case Action Subsystem5 : Subsystem  TreatAsAtomicUnit=on
  Switch Case Action Subsystem6 : Subsystem  TreatAsAtomicUnit=on
  Switch Case Action Subsystem7 : Subsystem  TreatAsAtomicUnit=on
  Switch Case Action Subsystem8 : Subsystem  TreatAsAtomicUnit=on
  Switch Case Action Subsystem9 : Subsystem  TreatAsAtomicUnit=on
  wires:
  Clock/1 -> Gain/1
  Switch Case/1 -> Switch Case Action Subsystem/Action
  Switch Case/2 -> Switch Case Action Subsystem1/Action
  Switch Case/3 -> Switch Case Action Subsystem2/Action
  Switch Case/10 -> Switch Case Action Subsystem3/Action
  Rounding Function/1 -> Switch Case/1
  In1/1 -> Switch Case Action Subsystem/1(In1), Switch Case Action Subsystem1/1(In1), Switch Case Action Subsystem2/1(In1), Switch Case Action Subsystem4/1(In1), Switch Case Action Subsystem5/1(In1), Switch Case Action Subsystem3/1(In1), Switch Case Action Subsystem9/1(In1), Switch Case Action Subsystem8/1(In1), Switch Case Action Subsystem7/1(In1), Switch Case Action Subsystem6/1(In1)
  Gain/1 -> Rounding Function/1
  Switch Case/4 -> Switch Case Action Subsystem4/Action
  Switch Case/5 -> Switch Case Action Subsystem5/Action
  Switch Case/6 -> Switch Case Action Subsystem6/Action
  Switch Case/7 -> Switch Case Action Subsystem7/Action
  Switch Case/8 -> Switch Case Action Subsystem8/Action
  Switch Case/9 -> Switch Case Action Subsystem9/Action

== system PNEUMA/Ventilator/Ventilator Controller ==
  note: Note that you will need to delete pulse block for your final controller design
  ABP : Inport
  SAO2 : Inport  Port=2
  Vt : Inport  Port=3
  BCO2 : Inport  Port=4
  Inspiratory O2 Partial Pressure : Subsystem  mask{begin_time=t_O2_start, end_time=t_O2_start+t_O2_duration, init_value=PIO2, final_value=PIO2+PIO2_change}
      mask prompts: begin_time "pulse begin"; end_time "pulse end"; init_value "initial value"; final_value "final value"
      mask Display: disp('pulse')
  Mean Arterial Pressure Estimation : Subsystem
  Mech Vent Pressure : Subsystem  mask{begin_time=t_Mech_Vent_start, end_time=t_Mech_Vent_start+t_Mech_Vent_duration, init_value=0, final_value=Mech_Vent_pressure}
      mask prompts: begin_time "pulse begin"; end_time "pulse end"; init_value "initial value"; final_value "final value"
      mask Display: disp('pulse')
  NM Block gain : Subsystem  mask{begin_time=t_NM_block_start, end_time=t_NM_block_start+t_NM_block_duration, NM_block_gain=NM_block_gain}
      mask prompts: begin_time "pulse begin"; end_time "pulse end"; NM_block_gain "neuromuscular block gain"
      mask Display: disp('pulse')
  Peak Breath CO2 Detector : Subsystem
  Peak Tidal Volume Detector : Subsystem
  Scope : Scope  NumInputPorts=2
  Scope1 : Scope
  Scope2 : Scope  NumInputPorts=2
  Scope3 : Scope  NumInputPorts=2
  Ventilator rate : Subsystem  mask{begin_time=t_Mech_Vent_start, end_time=t_Mech_Vent_start+t_Mech_Vent_duration, Ventilator_rate=Ventilator_rate}
      mask prompts: begin_time "pulse begin"; end_time "pulse end"; Ventilator_rate "ventilator rate"
      mask Display: disp('pulse')
  PIO2 : Outport
  NMB : Outport  Port=2
  VR : Outport  Port=3
  VP : Outport  Port=4
  wires:
  Mech Vent Pressure/1(Out1) -> VP/1
  Inspiratory O2 Partial Pressure/1(Out1) -> PIO2/1
  NM Block gain/1(Out1) -> NMB/1
  Ventilator rate/1(Out1) -> VR/1
  SAO2/1 -> Scope1/1
  Mean Arterial Pressure Estimation/1(MAP) -> Scope/2
  ABP/1 -> Scope/1, Mean Arterial Pressure Estimation/1(ABP)
  Vt/1 -> Peak Tidal Volume Detector/1(Vt), Scope2/1
  Peak Tidal Volume Detector/1(peakVt) -> Scope2/2
  BCO2/1 -> Scope3/1, Peak Breath CO2 Detector/1(BCO2)  "BCO2"
  Peak Breath CO2 Detector/1(peakBCO2) -> Scope3/2

== system PNEUMA/Cardiovascular System/Left Heart/Pmaxlv--Psa ---------------------- Rlv ==
  Pmax : Inport
  P : Inport  Port=2
  CHF Gain : Gain
  Gain : Gain  Gain=KRlv  SaturateOnIntegerOverflow=on  OutDataTypeStr=Inherit: Same as input  ParamDataTypeStr=Inherit: Same as input
  Product : Product  Inputs=/*  InputSameDT=on  RndMeth=Zero  SaturateOnIntegerOverflow=on  OutDataTypeStr=Inherit: Same as first input
  Saturation : Saturate  UpperLimit=inf  LowerLimit=0.01
  Flow : Outport
  wires:
  Pmax/1 -> CHF Gain/1
  Gain/1 -> Saturation/1
  P/1 -> Product/2
  Saturation/1 -> Product/1
  Product/1 -> Flow/1
  CHF Gain/1 -> Gain/1

== system PNEUMA/Cardiovascular System/Left Heart/Saving PVleft ==
  In1 : Inport
  Clock : Clock
  Gain : Gain  Gain=1/(3600*24*7)
  Rounding Function : Rounding
  Switch Case : SwitchCase  CaseConditions={0,1,2,3,4,5,6,7,8}  SampleTime=0.1
  Switch Case Action Subsystem : Subsystem  TreatAsAtomicUnit=on
  Switch Case Action Subsystem1 : Subsystem  TreatAsAtomicUnit=on
  Switch Case Action Subsystem2 : Subsystem  TreatAsAtomicUnit=on
  Switch Case Action Subsystem3 : Subsystem  TreatAsAtomicUnit=on
  Switch Case Action Subsystem4 : Subsystem  TreatAsAtomicUnit=on
  Switch Case Action Subsystem5 : Subsystem  TreatAsAtomicUnit=on
  Switch Case Action Subsystem6 : Subsystem  TreatAsAtomicUnit=on
  Switch Case Action Subsystem7 : Subsystem  TreatAsAtomicUnit=on
  Switch Case Action Subsystem8 : Subsystem  TreatAsAtomicUnit=on
  Switch Case Action Subsystem9 : Subsystem  TreatAsAtomicUnit=on
  wires:
  Clock/1 -> Gain/1
  Switch Case/1 -> Switch Case Action Subsystem/Action
  Switch Case/2 -> Switch Case Action Subsystem1/Action
  Switch Case/3 -> Switch Case Action Subsystem2/Action
  Switch Case/10 -> Switch Case Action Subsystem3/Action
  Rounding Function/1 -> Switch Case/1
  In1/1 -> Switch Case Action Subsystem/1(In1), Switch Case Action Subsystem1/1(In1), Switch Case Action Subsystem2/1(In1), Switch Case Action Subsystem5/1(In1), Switch Case Action Subsystem3/1(In1), Switch Case Action Subsystem9/1(In1), Switch Case Action Subsystem8/1(In1), Switch Case Action Subsystem7/1(In1), Switch Case Action Subsystem6/1(In1), Switch Case Action Subsystem4/1(In1)
  Gain/1 -> Rounding Function/1
  Switch Case/4 -> Switch Case Action Subsystem4/Action
  Switch Case/5 -> Switch Case Action Subsystem5/Action
  Switch Case/6 -> Switch Case Action Subsystem6/Action
  Switch Case/7 -> Switch Case Action Subsystem7/Action
  Switch Case/8 -> Switch Case Action Subsystem8/Action
  Switch Case/9 -> Switch Case Action Subsystem9/Action

== system PNEUMA/Cardiovascular System/Left Heart/SubSystem ==
  _ : Inport
  + : Inport  Port=2
  Saturation : Saturate  UpperLimit=10000  LowerLimit=0
  Sum : Sum  Inputs=|-+  InputSameDT=on  SaturateOnIntegerOverflow=on  OutDataTypeStr=Inherit: Same as first input
  Out : Outport
  wires:
  _/1 -> Sum/1
  +/1 -> Sum/2
  Sum/1 -> Saturation/1
  Saturation/1 -> Out/1

== system PNEUMA/Cardiovascular System/Left Heart/SubSystem1 ==
  _ : Inport
  + : Inport  Port=2
  Saturation : Saturate  UpperLimit=10000  LowerLimit=0
  Sum : Sum  Inputs=|-+  InputSameDT=on  SaturateOnIntegerOverflow=on  OutDataTypeStr=Inherit: Same as first input
  Out : Outport
  wires:
  Saturation/1 -> Out/1
  Sum/1 -> Saturation/1
  +/1 -> Sum/2
  _/1 -> Sum/1

== system PNEUMA/Cardiovascular System/Local Flow Regulation/Cerebral Circulation Regulation ==
  CaO2 : Inport
  PaCO2 : Inport  Port=2
  Qbp : Inport  Port=3
  Gsleep : Inport  Port=4
  " A+B/(1+C*exp(D*log10(PaCO2_n)))" : Constant  Value=48.6220
  1/tau_CO2 : Gain  Gain=1/tau_CO2
  1/tau_O2 : Gain  Gain=1/tau_O2
  C : Gain  Gain=C
  Constant : Constant
  Constant1 : Constant
  Constant2 : Constant
  Constant3 : Constant  Value=B
  Constant4 : Constant  Value=A
  CvbO2_n : Constant  Value=CvbO2_n
  D : Gain  Gain=D
  Divide : Product  Inputs=*/
  Divide1 : Product  Inputs=*/
  Divide2 : Product  Inputs=/*/
  Divide3 : Product  Inputs=*/
  GbO2 : Gain  Gain=GbO2
  Gbpn : Gain  Gain=1/Rbpn
  Integrator : Integrator
  Integrator1 : Integrator
  Math Function : Math  Operator=log10  SignedPower=on
  Math Function1 : Math  SignedPower=on
  Mb : Constant  Value=Mb
  Subsystem : Subsystem
  Subtract : Sum  Inputs=+--
  Subtract1 : Sum  Inputs=--
  Subtract2 : Sum  Inputs=+++
  Subtract3 : Sum  Inputs=--+
  Sum : Sum  Inputs=|++
  Sum1 : Sum  Inputs=|++
  Gbp : Outport
  wires:
  Mb/1 -> Divide/1
  Divide/1 -> Subtract/2
  CvbO2_n/1 -> Subtract/3
  Subtract/1 -> Divide3/1
  GbO2/1 -> Subtract1/2
  Subtract1/1 -> 1/tau_O2/1
  1/tau_O2/1 -> Integrator/1
  Integrator/1 -> Subtract1/1, Subtract2/2
  Constant/1 -> Subtract2/1
  1/tau_CO2/1 -> Integrator1/1
  Integrator1/1 -> Subtract2/3, Subtract3/1
  Subtract3/1 -> 1/tau_CO2/1
  Constant1/1 -> Subtract3/2
  Math Function/1 -> D/1
  D/1 -> Math Function1/1
  Math Function1/1 -> C/1
  C/1 -> Sum/1
  Constant2/1 -> Sum/2
  Constant3/1 -> Divide1/1
  Sum/1 -> Divide1/2
  Divide1/1 -> Sum1/1
  Constant4/1 -> Sum1/2
  Sum1/1 -> Divide2/2
  " A+B/(1+C*exp(D*log10(PaCO2_n)))"/1 -> Divide2/3
  Divide2/1 -> Subtract3/3
  Gbpn/1 -> Gbp/1
  CaO2/1 -> Subtract/1
  PaCO2/1 -> Math Function/1
  Subtract2/1 -> Gbpn/1
  Qbp/1 -> Subsystem/1(QbpIC)
  Subsystem/1(Qbp) -> Divide/2
  Gsleep/1 -> Divide3/2, Divide2/1
  Divide3/1 -> GbO2/1

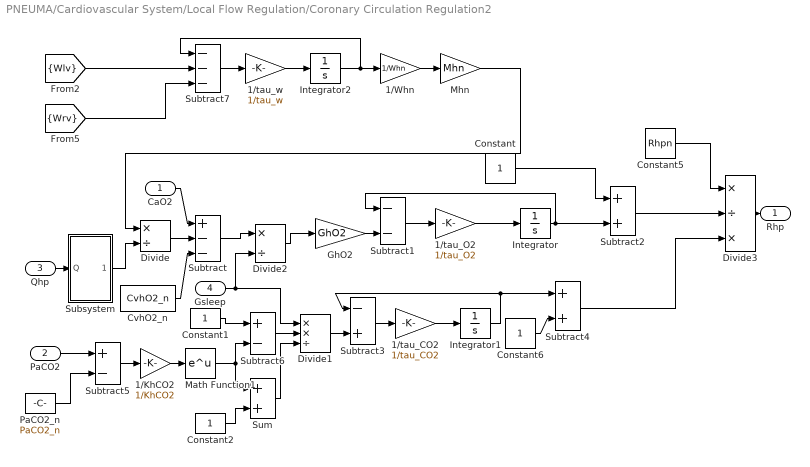
== system PNEUMA/Cardiovascular System/Local Flow Regulation/Coronary Circulation Regulation2 ==
  CaO2 : Inport
  PaCO2 : Inport  Port=2
  Qhp : Inport  Port=3
  Gsleep : Inport  Port=4
  1/KhCO2 : Gain  Gain=1/KhCO2
  1/Whn : Gain  Gain=1/Whn
  1/tau_CO2 : Gain  Gain=1/tau_CO2
  1/tau_O2 : Gain  Gain=1/tau_O2
  1/tau_w : Gain  Gain=1/tau_w
  Constant{,1..2,6} (4 alike) : Constant
  Constant5 : Constant  Value=Rhpn
  CvhO2_n : Constant  Value=CvhO2_n
  Divide : Product  Inputs=*/
  Divide1 : Product  Inputs=**/
  Divide2 : Product  Inputs=*/
  Divide3 : Product  Inputs=*/*
  GhO2 : Gain  Gain=GhO2
  Integrator : Integrator
  Integrator1 : Integrator
  Integrator2 : Integrator
  Math Function1 : Math  SignedPower=on
  Mhn : Gain  Gain=Mhn
  PaCO2_n : Constant  Value=PaCO2_n
  Subsystem : Subsystem
  Subtract : Sum  Inputs=+--
  Subtract1 : Sum  Inputs=--
  Subtract2 : Sum
  Subtract3 : Sum  Inputs=-+
  Subtract4 : Sum
  Subtract5 : Sum  Inputs=+-
  Subtract6 : Sum  Inputs=+-
  Subtract7 : Sum  Inputs=---
  Sum : Sum
  Rhp : Outport
  wires:
  Divide/1 -> Subtract/2
  CvhO2_n/1 -> Subtract/3
  GhO2/1 -> Subtract1/2
  Subtract1/1 -> 1/tau_O2/1
  1/tau_O2/1 -> Integrator/1
  Integrator/1 -> Subtract1/1, Subtract2/2
  Constant/1 -> Subtract2/1
  1/tau_CO2/1 -> Integrator1/1
  Integrator1/1 -> Subtract3/1, Subtract4/1
  Subtract3/1 -> 1/tau_CO2/1
  Subtract5/1 -> 1/KhCO2/1
  1/KhCO2/1 -> Math Function1/1
  Math Function1/1 -> Subtract6/2, Sum/1
  Constant2/1 -> Sum/2
  Subtract6/1 -> Divide1/2
  Sum/1 -> Divide1/3
  Constant5/1 -> Divide3/1
  Subtract2/1 -> Divide3/2
  Divide3/1 -> Rhp/1
  CaO2/1 -> Subtract/1
  PaCO2/1 -> Subtract5/1
  Constant6/1 -> Subtract4/2
  Subtract4/1 -> Divide3/3
  PaCO2_n/1 -> Subtract5/2
  Constant1/1 -> Subtract6/1
  Divide1/1 -> Subtract3/2
  1/tau_w/1 -> Integrator2/1
  Subtract7/1 -> 1/tau_w/1
  Integrator2/1 -> 1/Whn/1, Subtract7/1
  1/Whn/1 -> Mhn/1
  [Wlv] -> Subtract7/2
  [Wrv] -> Subtract7/3
  Subsystem/1(Qhp) -> Divide/2
  Qhp/1 -> Subsystem/1(Q)
  Mhn/1 -> Divide/1
  Gsleep/1 -> Divide2/2, Divide1/1
  Subtract/1 -> Divide2/1
  Divide2/1 -> GhO2/1

== system PNEUMA/Cardiovascular System/Local Flow Regulation/Muscular Circulation Regulation1 ==
  CaO2 : Inport
  PaCO2 : Inport  Port=2
  Qmp : Inport  Port=3
  Gsleep : Inport  Port=4
  1/KmCO2 : Gain  Gain=1/KmCO2
  1/tau_CO2 : Gain  Gain=1/tau_CO2
  1/tau_O2 : Gain  Gain=1/tau_O2
  Constant{,1..2,6} (4 alike) : Constant
  CvmO2_n : Constant  Value=CvmO2_n
  Divide : Product  Inputs=*/
  Divide1 : Product  Inputs=**/
  Divide2 : Product  Inputs=*/
  Divide3 : Product  Inputs=*/*
  GmO2 : Gain  Gain=GmO2
  Integrator : Integrator  LimitOutput=on  UpperSaturationLimit=10000  LowerSaturationLimit=0
  Integrator1 : Integrator
  Math Function1 : Math  SignedPower=on
  Mm : Constant  Value=Mm
  PaCO2_n : Constant  Value=PaCO2_n
  Subsystem : Subsystem
  Subtract : Sum  Inputs=+--
  Subtract1 : Sum  Inputs=--
  Subtract2 : Sum
  Subtract3 : Sum  Inputs=-+
  Subtract4 : Sum
  Subtract5 : Sum  Inputs=+-
  Subtract6 : Sum  Inputs=+-
  Sum : Sum
  Rmp : Outport
  wires:
  Mm/1 -> Divide/1
  Divide/1 -> Subtract/2
  CvmO2_n/1 -> Subtract/3
  GmO2/1 -> Subtract1/2
  Subtract1/1 -> 1/tau_O2/1
  1/tau_O2/1 -> Integrator/1
  Integrator/1 -> Subtract1/1, Subtract2/2
  Constant/1 -> Subtract2/1
  1/tau_CO2/1 -> Integrator1/1
  Integrator1/1 -> Subtract3/1, Subtract4/1
  Subtract3/1 -> 1/tau_CO2/1
  Subtract5/1 -> 1/KmCO2/1
  1/KmCO2/1 -> Math Function1/1
  Math Function1/1 -> Subtract6/2, Sum/1
  Constant2/1 -> Sum/2
  Subtract6/1 -> Divide1/2
  Sum/1 -> Divide1/3
  [Rmpn] -> Divide3/1
  Subtract2/1 -> Divide3/2
  Divide3/1 -> Rmp/1
  CaO2/1 -> Subtract/1
  PaCO2/1 -> Subtract5/1
  Constant6/1 -> Subtract4/2
  Subtract4/1 -> Divide3/3
  PaCO2_n/1 -> Subtract5/2
  Constant1/1 -> Subtract6/1
  Divide1/1 -> Subtract3/2
  Qmp/1 -> Subsystem/1(Q)
  Subsystem/1(Qmp) -> Divide/2
  Subtract/1 -> Divide2/1
  Gsleep/1 -> Divide2/2, Divide1/1
  Divide2/1 -> GmO2/1

== system PNEUMA/Cardiovascular System/Pulmonary/SubSystem ==
  _ : Inport
  + : Inport  Port=2
  Saturation : Saturate  UpperLimit=10000  LowerLimit=0
  Sum : Sum  Inputs=|-+  InputSameDT=on  SaturateOnIntegerOverflow=on  OutDataTypeStr=Inherit: Same as first input
  Out : Outport
  wires:
  _/1 -> Sum/1
  +/1 -> Sum/2
  Sum/1 -> Saturation/1
  Saturation/1 -> Out/1

== system PNEUMA/Cardiovascular System/Pulmonary/SubSystem1 ==
  _ : Inport
  + : Inport  Port=2
  Saturation : Saturate  UpperLimit=10000  LowerLimit=0
  Sum : Sum  Inputs=|-+  InputSameDT=on  SaturateOnIntegerOverflow=on  OutDataTypeStr=Inherit: Same as first input
  Out : Outport
  wires:
  _/1 -> Sum/1
  +/1 -> Sum/2
  Sum/1 -> Saturation/1
  Saturation/1 -> Out/1

== system PNEUMA/Cardiovascular System/Pulmonary/SubSystem2 ==
  _ : Inport
  + : Inport  Port=2
  Saturation : Saturate  UpperLimit=10000  LowerLimit=0
  Sum : Sum  Inputs=|-+  InputSameDT=on  SaturateOnIntegerOverflow=on  OutDataTypeStr=Inherit: Same as first input
  Out : Outport
  wires:
  Saturation/1 -> Out/1
  Sum/1 -> Saturation/1
  +/1 -> Sum/2
  _/1 -> Sum/1

== system PNEUMA/Cardiovascular System/Right Heart/Pmaxrv--Ppa ---------------------- Rrv ==
  Pmax : Inport
  P : Inport  Port=2
  Gain : Gain  Gain=KRrv  SaturateOnIntegerOverflow=on  OutDataTypeStr=Inherit: Same as input  ParamDataTypeStr=Inherit: Same as input
  Product : Product  Inputs=/*  InputSameDT=on  RndMeth=Zero  SaturateOnIntegerOverflow=on  OutDataTypeStr=Inherit: Same as first input
  Saturation : Saturate  UpperLimit=inf  LowerLimit=0.01
  Flow : Outport
  wires:
  Pmax/1 -> Gain/1
  Gain/1 -> Saturation/1
  P/1 -> Product/2
  Saturation/1 -> Product/1
  Product/1 -> Flow/1

== system PNEUMA/Cardiovascular System/Right Heart/SubSystem ==
  _ : Inport
  + : Inport  Port=2
  Saturation : Saturate  UpperLimit=10000  LowerLimit=0
  Sum : Sum  Inputs=|-+  InputSameDT=on  SaturateOnIntegerOverflow=on  OutDataTypeStr=Inherit: Same as first input
  Out : Outport
  wires:
  _/1 -> Sum/1
  +/1 -> Sum/2
  Sum/1 -> Saturation/1
  Saturation/1 -> Out/1

== system PNEUMA/Cardiovascular System/Right Heart/SubSystem1 ==
  _ : Inport
  + : Inport  Port=2
  Saturation : Saturate  UpperLimit=10000  LowerLimit=0
  Sum : Sum  Inputs=|-+  InputSameDT=on  SaturateOnIntegerOverflow=on  OutDataTypeStr=Inherit: Same as first input
  Out : Outport
  wires:
  Saturation/1 -> Out/1
  Sum/1 -> Saturation/1
  +/1 -> Sum/2
  _/1 -> Sum/1

== system PNEUMA/Cardiovascular System/SA-node and Autonomic Control/Heart Emaxlv ==
  ftbs : Inport
  Gbs(SI) : Inport  Port=2
  Basal_Emaxlv : Constant  Value=2.392
  Constant : Constant  Value=ftbs_min
  Gain_Emaxlv : Gain  Gain=0.475  SaturateOnIntegerOverflow=on  OutDataTypeStr=Inherit: Same as input  ParamDataTypeStr=Inherit: Same as input
  Math Function : Math  Operator=log  SignedPower=on
  Product3 : Product  InputSameDT=on  SaturateOnIntegerOverflow=on  OutDataTypeStr=Inherit: Same as first input
  Saturation : Saturate  UpperLimit=inf  LowerLimit=1
  Sum : Sum  Inputs=+-  InputSameDT=on  SaturateOnIntegerOverflow=on  OutDataTypeStr=Inherit: Same as first input
  Sum1 : Sum  InputSameDT=on  SaturateOnIntegerOverflow=on  OutDataTypeStr=Inherit: Same as first input
  Transfer Fcn : TransferFcn  Denominator=[toux(1) 1]
  Transport Delay : TransportDelay  DelayTime=Dx(1)  BufferSize=19456
  Emaxlv : Outport
  wires:
  ftbs/1 -> Transport Delay/1
  Transport Delay/1 -> Sum/1
  Constant/1 -> Sum/2
  Sum/1 -> Saturation/1
  Saturation/1 -> Math Function/1
  Math Function/1 -> Gain_Emaxlv/1
  Transfer Fcn/1 -> Sum1/1
  Sum1/1 -> Emaxlv/1
  Basal_Emaxlv/1 -> Sum1/2
  Gbs(SI)/1 -> Product3/2
  Gain_Emaxlv/1 -> Product3/1
  Product3/1 -> Transfer Fcn/1
